simulink model "mathemeticalModel"  (R2018a)
settings: Solver=VariableStepAuto  StartTime=0.0  StopTime=15/ffund  RelTol=1e-3
values from neighbouring files (symbols this model uses):
  ffund = 50    [InverterMFile.m]    (also in mathematicalModelParam.m; sim_param_new_board.m)
  La = 3.4e-9+1.3e-9+2.02e-8    (= 2.49e-08)    [mathematicalModelParam.m]
  Lload = 6.9e-3    (= 0.0069)    [mathematicalModelParam.m]
  ModulationIndex = 0.9    [mathematicalModelParam.m]
  Ra = 2.02e-8+3.4e-9+1.3e-9    (= 2.49e-08)    [mathematicalModelParam.m]
  Rload = 10    [mathematicalModelParam.m]
  Vdc = Vmodule*series    (= 270)    [InverterMFile.m]    (also in mathematicalModelParam.m; sim_param_new_board.m)
libraries: powerlib_meascontrol x6, simulink x3
settings Model: Creator=enes_  LastModifiedBy=enes_

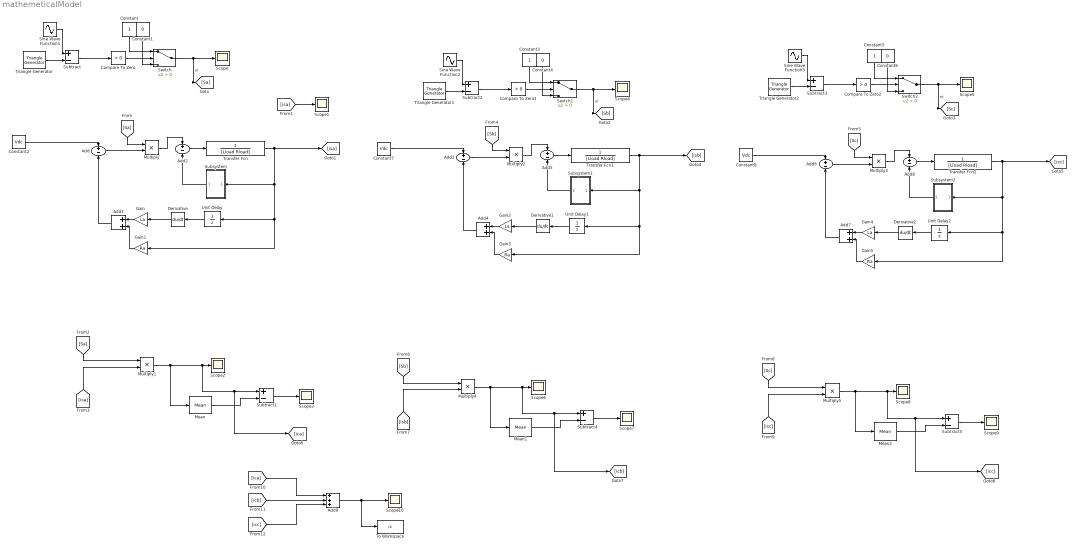
== system mathemeticalModel ==
  Add{,2..3,5..6,8} (6 alike) : Sum  Inputs=+-
  Add1 : Sum
  Add4 : Sum
  Add7 : Sum
  Add9 : Sum  Inputs=+++
  Compare To Zero : simulink/Logic and Bit Operations/Compare To Zero  relop=>  OutDataTypeStr=boolean
  Compare To Zero1 : simulink/Logic and Bit Operations/Compare To Zero  relop=>  OutDataTypeStr=boolean
  Compare To Zero2 : simulink/Logic and Bit Operations/Compare To Zero  relop=>  OutDataTypeStr=boolean
  Constant : Constant
  Constant1 : Constant  Value=0
  Constant2 : Constant  Value=Vdc
  Constant3 : Constant
  Constant4 : Constant  Value=0
  Constant5 : Constant
  Constant6 : Constant  Value=0
  Constant7 : Constant  Value=Vdc
  Constant8 : Constant  Value=Vdc
  Derivative : Derivative
  Derivative1 : Derivative
  Derivative2 : Derivative
  Gain : Gain  Gain=La
  Gain1 : Gain  Gain=Ra
  Gain2 : Gain  Gain=La
  Gain3 : Gain  Gain=Ra
  Gain4 : Gain  Gain=La
  Gain5 : Gain  Gain=Ra
  Mean : powerlib_meascontrol/Measurements/Mean  Freq=ffund  Vinit=0  Ts=0
  Mean1 : powerlib_meascontrol/Measurements/Mean  Freq=ffund  Vinit=0  Ts=0
  Mean2 : powerlib_meascontrol/Measurements/Mean  Freq=ffund  Vinit=0  Ts=0
  Multiply{,1..5} (6 alike) : Product
  Scope{,1..10} (11 alike) : Scope
  Sine Wave Function1 : Sin  Amplitude=ModulationIndex  Frequency=ffund*2*pi  SampleTime=0
  Sine Wave Function2 : Sin  Amplitude=ModulationIndex  Frequency=ffund*2*pi  Phase=-120  SampleTime=0
  Sine Wave Function3 : Sin  Amplitude=ModulationIndex  Frequency=ffund*2*pi  Phase=-120  SampleTime=0
  Subsystem : Subsystem
  Subsystem1 : Subsystem
  Subsystem2 : Subsystem
  Subtract{,1..5} (6 alike) : Sum  Inputs=+-
  Switch : Switch  Criteria=u2 > Threshold
  Switch1 : Switch  Criteria=u2 > Threshold
  Switch2 : Switch  Criteria=u2 > Threshold
  To Workspace : ToWorkspace  VariableName=ic  SaveFormat=Timeseries  SampleTime=-1
  Transfer Fcn : TransferFcn  Denominator=[Lload Rload]
  Transfer Fcn1 : TransferFcn  Denominator=[Lload Rload]
  Transfer Fcn2 : TransferFcn  Denominator=[Lload Rload]
  Triangle Generator : powerlib_meascontrol/Pulse & Signal Generators/Triangle Generator  Freq=fsw  Phase=0  Ts=0
  Triangle Generator1 : powerlib_meascontrol/Pulse & Signal Generators/Triangle Generator  Freq=fsw  Phase=0  Ts=0
  Triangle Generator2 : powerlib_meascontrol/Pulse & Signal Generators/Triangle Generator  Freq=fsw  Phase=120  Ts=0
  Unit Delay : UnitDelay  SampleTime=-1
  Unit Delay1 : UnitDelay  SampleTime=-1
  Unit Delay2 : UnitDelay  SampleTime=-1
  wires:
  Subtract/1 -> Compare To Zero/1
  Triangle Generator/1 -> Subtract/2
  Sine Wave Function1/1 -> Subtract/1
  Constant/1 -> Switch/1
  Compare To Zero/1 -> Switch/2
  Constant1/1 -> Switch/3
  Switch/1 -> [Sa], Scope/1  "at"
  Constant2/1 -> Add/1
  Unit Delay/1 -> Derivative/1
  Add/1 -> Multiply/2
  [Sa] -> Multiply/1
  Transfer Fcn/1 -> [isa], Subsystem/1(In1), Gain1/1, Unit Delay/1
  [isa] -> Scope1/1
  Derivative/1 -> Gain/1
  [Sa] -> Multiply1/1
  [isa] -> Multiply1/2
  Multiply1/1 -> Mean/1, [ica], Subtract1/1, Scope2/1
  Mean/1 -> Subtract1/2
  Gain/1 -> Add1/1
  Add1/1 -> Add/2
  Gain1/1 -> Add1/2
  Add2/1 -> Transfer Fcn/1
  Multiply/1 -> Add2/1
  Subsystem/1(Out1) -> Add2/2
  Subtract1/1 -> Scope3/1
  Constant4/1 -> Switch1/3
  Switch1/1 -> [Sb], Scope4/1  "at"
  Sine Wave Function2/1 -> Subtract2/1
  Subtract2/1 -> Compare To Zero1/1
  Triangle Generator1/1 -> Subtract2/2
  Constant3/1 -> Switch1/1
  Compare To Zero1/1 -> Switch1/2
  Constant5/1 -> Switch2/1
  Triangle Generator2/1 -> Subtract3/2
  Switch2/1 -> [Sc], Scope5/1  "at"
  Subtract3/1 -> Compare To Zero2/1
  Sine Wave Function3/1 -> Subtract3/1
  Constant6/1 -> Switch2/3
  Compare To Zero2/1 -> Switch2/2
  Gain2/1 -> Add4/1
  Gain3/1 -> Add4/2
  Derivative1/1 -> Gain2/1
  Unit Delay1/1 -> Derivative1/1
  Constant7/1 -> Add3/1
  Multiply2/1 -> Add5/1
  Subsystem1/1(Out1) -> Add5/2
  Add3/1 -> Multiply2/2
  Add4/1 -> Add3/2
  [Sb] -> Multiply2/1
  Transfer Fcn1/1 -> [isb], Subsystem1/1(In1), Gain3/1, Unit Delay1/1
  Add5/1 -> Transfer Fcn1/1
  Gain4/1 -> Add7/1
  Gain5/1 -> Add7/2
  Derivative2/1 -> Gain4/1
  Unit Delay2/1 -> Derivative2/1
  Constant8/1 -> Add6/1
  Multiply3/1 -> Add8/1
  Subsystem2/1(Out1) -> Add8/2
  Add6/1 -> Multiply3/2
  Add7/1 -> Add6/2
  [Sc] -> Multiply3/1
  Transfer Fcn2/1 -> [isc], Subsystem2/1(In1), Gain5/1, Unit Delay2/1
  Add8/1 -> Transfer Fcn2/1
  Mean1/1 -> Subtract4/2
  Multiply4/1 -> Mean1/1, [icb], Subtract4/1, Scope6/1
  [isb] -> Multiply4/2
  Subtract4/1 -> Scope7/1
  [Sb] -> Multiply4/1
  Mean2/1 -> Subtract5/2
  Multiply5/1 -> Mean2/1, [icc], Subtract5/1, Scope8/1
  [isc] -> Multiply5/2
  Subtract5/1 -> Scope9/1
  [Sc] -> Multiply5/1
  [ica] -> Add9/1
  [icb] -> Add9/2
  [icc] -> Add9/3
  Add9/1 -> To Workspace/1, Scope10/1

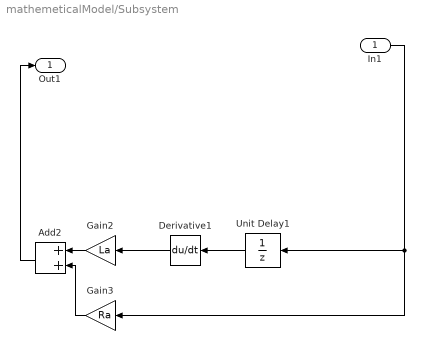
== system mathemeticalModel/Subsystem ==
  In1 : Inport
  Add2 : Sum
  Derivative1 : Derivative
  Gain2 : Gain  Gain=La
  Gain3 : Gain  Gain=Ra
  Unit Delay1 : UnitDelay  SampleTime=-1
  Out1 : Outport
  wires:
  Derivative1/1 -> Gain2/1
  Unit Delay1/1 -> Derivative1/1
  In1/1 -> Gain3/1, Unit Delay1/1
  Gain2/1 -> Add2/1
  Gain3/1 -> Add2/2
  Add2/1 -> Out1/1

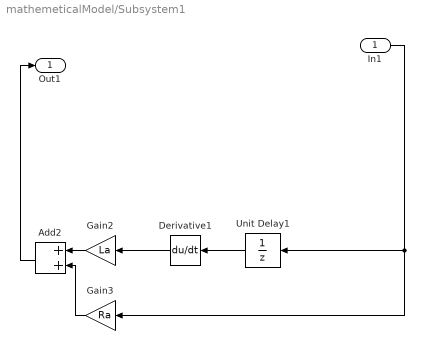
== system mathemeticalModel/Subsystem1 ==
  In1 : Inport
  Add2 : Sum
  Derivative1 : Derivative
  Gain2 : Gain  Gain=La
  Gain3 : Gain  Gain=Ra
  Unit Delay1 : UnitDelay  SampleTime=-1
  Out1 : Outport
  wires:
  Derivative1/1 -> Gain2/1
  Unit Delay1/1 -> Derivative1/1
  In1/1 -> Gain3/1, Unit Delay1/1
  Gain2/1 -> Add2/1
  Gain3/1 -> Add2/2
  Add2/1 -> Out1/1

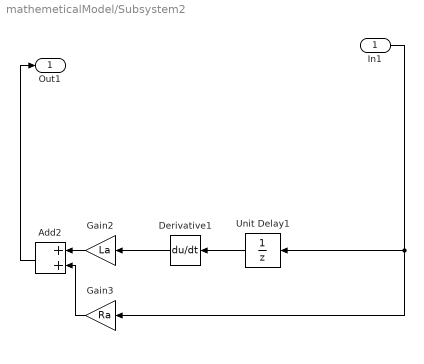
== system mathemeticalModel/Subsystem2 ==
  In1 : Inport
  Add2 : Sum
  Derivative1 : Derivative
  Gain2 : Gain  Gain=La
  Gain3 : Gain  Gain=Ra
  Unit Delay1 : UnitDelay  SampleTime=-1
  Out1 : Outport
  wires:
  Derivative1/1 -> Gain2/1
  Unit Delay1/1 -> Derivative1/1
  In1/1 -> Gain3/1, Unit Delay1/1
  Gain2/1 -> Add2/1
  Gain3/1 -> Add2/2
  Add2/1 -> Out1/1
